simulink subsystem "Diffusion"  (R2022a)
settings: Solver=VariableStepAuto  StartTime=0.0  StopTime=10.0  RelTol=1e-3
undefined symbols (not defined in the file or in its folder): alfa, beta, Cn, vocFitSimulink
settings Model: Creator=mateu  LastModifiedBy=mmarq

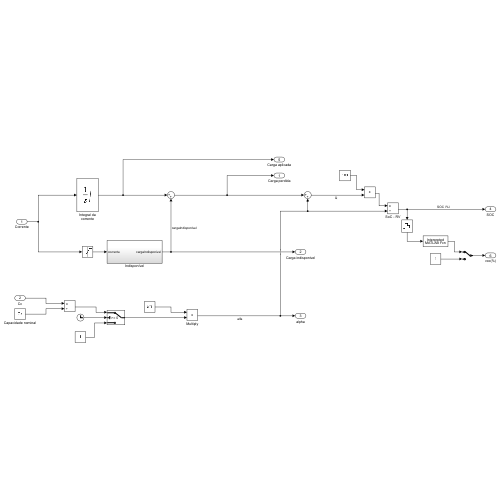
[thumbnail: Simulink's stored preview of the top-level diagram]
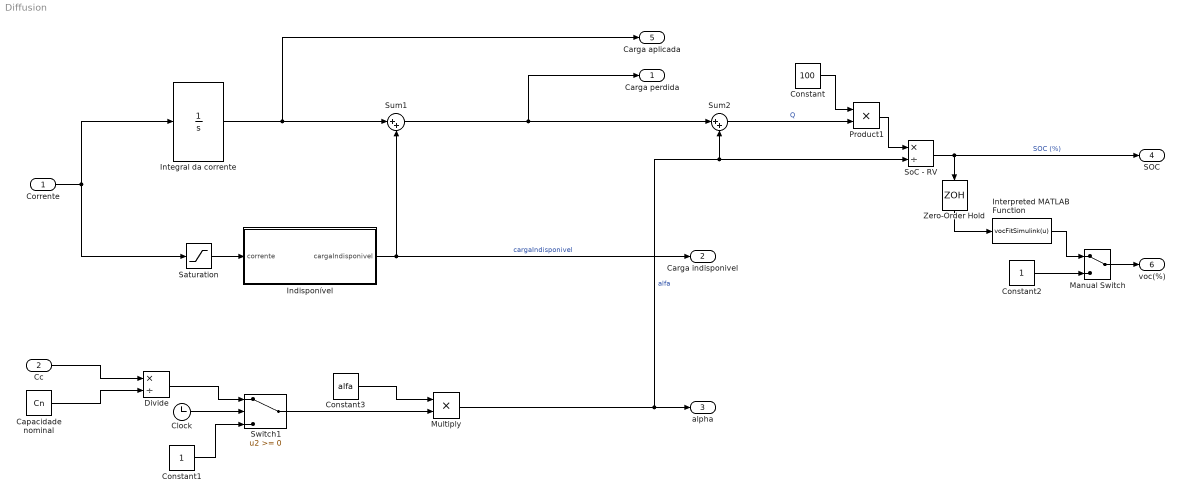
== system Diffusion ==
  Corrente : Inport
  Cc : Inport  Port=2
  Capacidade nominal : Constant  Value=Cn
  Clock : Clock
  Constant : Constant  Value=100
  Constant1 : Constant
  Constant2 : Constant
  Constant3 : Constant  Value=alfa
  Divide : Product  Inputs=*/
  Indisponível : Subsystem
  Integral da corrente : Integrator  LimitOutput=on  UpperSaturationLimit=0  LowerSaturationLimit=-alfa
  Interpreted MATLAB Function : MATLABFcn  MATLABFcn=vocFitSimulink(u)
  Manual Switch : ManualSwitch
  Multiply : Product
  Product1 : Product
  Saturation : Saturate  UpperLimit=0  LowerLimit=-Inf
  SoC - RV : Product  Inputs=*/
  Sum1 : Sum  Inputs=|++
  Sum2 : Sum  Inputs=|++
  Switch1 : Switch  SaturateOnIntegerOverflow=off  InputSameDT=off
  Zero-Order Hold : ZeroOrderHold  SampleTime=0.1
  Carga perdida : Outport  VectorParamsAs1DForOutWhenUnconnected=off
  Carga indisponivel : Outport  Port=2  VectorParamsAs1DForOutWhenUnconnected=off
  alpha : Outport  Port=3  VectorParamsAs1DForOutWhenUnconnected=off
  SOC : Outport  Port=4
  Carga aplicada : Outport  Port=5  VectorParamsAs1DForOutWhenUnconnected=off
  voc(%) : Outport  Port=6
  wires:
  Manual Switch/1 -> voc(%)/1
  Corrente/1 -> Saturation/1, Integral da corrente/1
  Cc/1 -> Divide/1
  Clock/1 -> Switch1/2
  Sum1/1 -> Sum2/1, Carga perdida/1
  Constant2/1 -> Manual Switch/2
  Integral da corrente/1 -> Sum1/1, Carga aplicada/1
  Capacidade nominal/1 -> Divide/2
  Divide/1 -> Switch1/1
  Constant3/1 -> Multiply/1
  Multiply/1 -> alpha/1, SoC - RV/2, Sum2/2  "alfa"
  Constant1/1 -> Switch1/3
  Sum2/1 -> Product1/2  "Q"
  Product1/1 -> SoC - RV/1
  Constant/1 -> Product1/1
  Indisponível/1(cargaIndisponivel) -> Carga indisponivel/1, Sum1/2  "cargaIndisponivel"
  Zero-Order Hold/1 -> Interpreted MATLAB Function/1
  Saturation/1 -> Indisponível/1(corrente)
  Interpreted MATLAB Function/1 -> Manual Switch/1
  SoC - RV/1 -> SOC/1, Zero-Order Hold/1  "SOC (%)"
  Switch1/1 -> Multiply/2

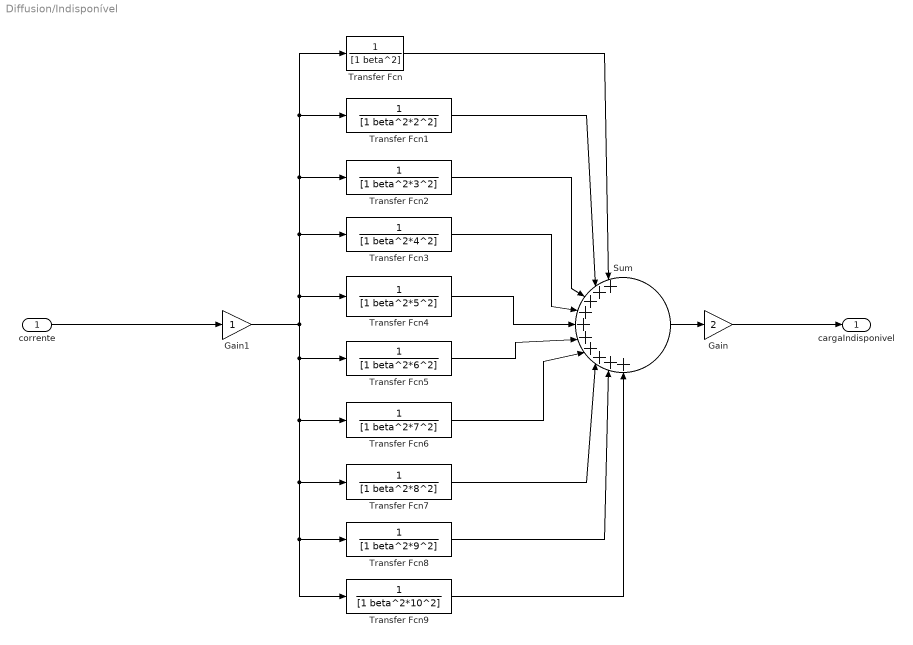
== system Diffusion/Indisponível ==
  corrente : Inport
  Gain : Gain  Gain=2
  Gain1 : Gain
  Sum : Sum  Inputs=|++++++++++
  Transfer Fcn : TransferFcn  Denominator=[1 beta^2]
  Transfer Fcn1 : TransferFcn  Denominator=[1 beta^2*2^2]
  Transfer Fcn2 : TransferFcn  Denominator=[1 beta^2*3^2]
  Transfer Fcn3 : TransferFcn  Denominator=[1 beta^2*4^2]
  Transfer Fcn4 : TransferFcn  Denominator=[1 beta^2*5^2]
  Transfer Fcn5 : TransferFcn  Denominator=[1 beta^2*6^2]
  Transfer Fcn6 : TransferFcn  Denominator=[1 beta^2*7^2]
  Transfer Fcn7 : TransferFcn  Denominator=[1 beta^2*8^2]
  Transfer Fcn8 : TransferFcn  Denominator=[1 beta^2*9^2]
  Transfer Fcn9 : TransferFcn  Denominator=[1 beta^2*10^2]
  cargaIndisponivel : Outport  VectorParamsAs1DForOutWhenUnconnected=off
  wires:
  Gain/1 -> cargaIndisponivel/1
  corrente/1 -> Gain1/1
  Gain1/1 -> Transfer Fcn/1, Transfer Fcn1/1, Transfer Fcn2/1, Transfer Fcn3/1, Transfer Fcn4/1, Transfer Fcn9/1, Transfer Fcn8/1, Transfer Fcn7/1, Transfer Fcn6/1, Transfer Fcn5/1
  Sum/1 -> Gain/1
  Transfer Fcn9/1 -> Sum/10
  Transfer Fcn8/1 -> Sum/9
  Transfer Fcn7/1 -> Sum/8
  Transfer Fcn6/1 -> Sum/7
  Transfer Fcn5/1 -> Sum/6
  Transfer Fcn4/1 -> Sum/5
  Transfer Fcn3/1 -> Sum/4
  Transfer Fcn2/1 -> Sum/3
  Transfer Fcn1/1 -> Sum/2
  Transfer Fcn/1 -> Sum/1
